simulink model "transferfunctiondisturbance5"  (R2021b)
settings: Solver=ode23s  StartTime=0.0  StopTime=1000  RelTol=1e-3
settings Model: Creator=User  LastModifiedBy=User

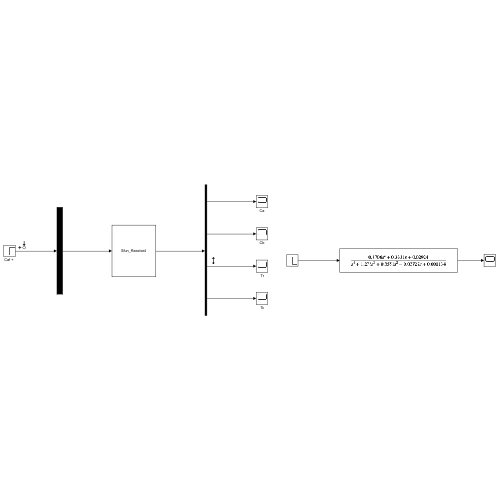
[thumbnail: Simulink's stored preview of the top-level diagram]
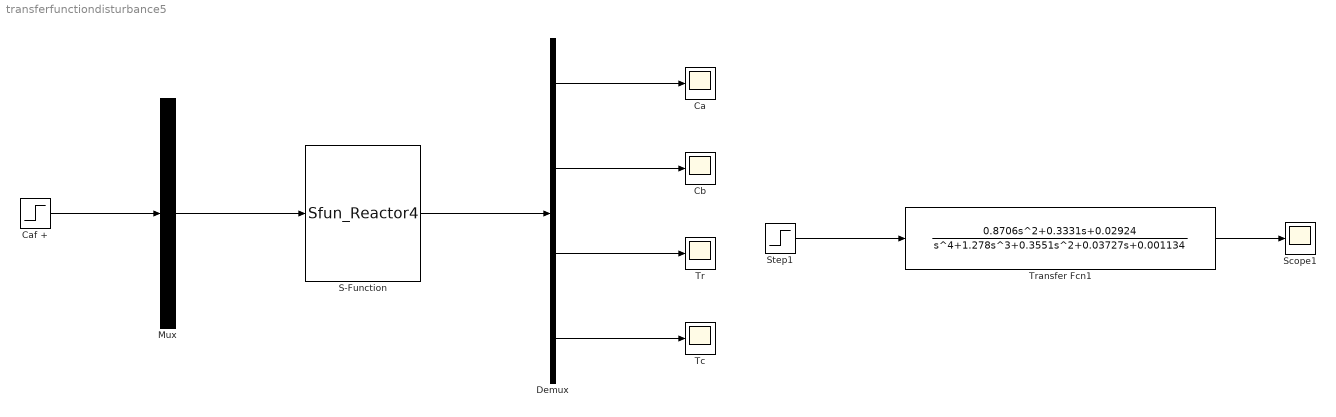
== system transferfunctiondisturbance5 ==
  " Tc" : Scope
  " Tr" : Scope
  Ca : Scope
  "Caf + " : Step  Time=0  Before=2.85  After=2.9925  SampleTime=0
  Cb : Scope
  Demux : Demux
  Mux : Mux  Inputs=1
  S-Function : S-Function  FunctionName=Sfun_Reactor4  SFunctionDeploymentMode=off  EnableBusSupport=off
  Scope1 : Scope
  Step1 : Step  Time=0  After=-0.1425  SampleTime=0
  Transfer Fcn1 : TransferFcn  Numerator=[0.8706 0.3331 0.02924]  Denominator=[1 1.278 0.3551 0.03727 0.001134]
  wires:
  "Caf + "/1 -> Mux/1
  Demux/1 -> Ca/1
  Demux/3 -> " Tr"/1
  Demux/2 -> Cb/1
  Demux/4 -> " Tc"/1
  S-Function/1 -> Demux/1
  Mux/1 -> S-Function/1
  Transfer Fcn1/1 -> Scope1/1
  Step1/1 -> Transfer Fcn1/1
